simulink model "sistemaUno"  (R2013b)
settings: Solver=ode45  StartTime=0.0  StopTime=100  RelTol=1e-5
settings Model: Creator=juan_  LastModifiedBy=juan_

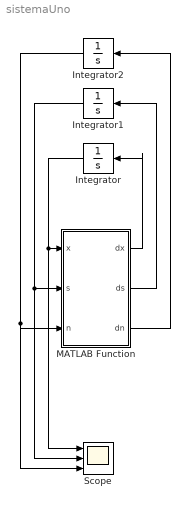
== system sistemaUno ==
  Integrator : Integrator  InitialCondition=1
  Integrator1 : Integrator  InitialCondition=50
  Integrator2 : Integrator  InitialCondition=10
  MATLAB Function : MATLAB Function  TreatAsAtomicUnit=on
  Scope : Scope  NumInputPorts=3
      settings: TimeRange=50  YMin=-5~-5~-5  YMax=5~5~5  SampleInput=on
  wires:
  MATLAB Function/1(dx) -> Integrator/1
  Integrator/1 -> Scope/1, MATLAB Function/1(x)
  MATLAB Function/2(ds) -> Integrator1/1
  MATLAB Function/3(dn) -> Integrator2/1
  Integrator1/1 -> Scope/2, MATLAB Function/2(s)
  Integrator2/1 -> Scope/3, MATLAB Function/3(n)

== matlab function sistemaUno/MATLAB Function ==
  data: x input; dx output; s input; n input; ds output; dn output
function [dx,ds,dn] = fcn(x,s,n)

k1=1/0.45;
k2=0.108;
s_in=50;
n_in=5;
D=0;

x0=1;
s0=50;
n0=10;

mu_max=0.5;
Ks=0.5;
rx=x*mu_max*s/(Ks+s);
rs=-k1*rx;
rn=-k2*rx;

dx= rx+D*(-x);
ds= rs+D*(s_in-s);
dn= rn+D*(n_in-n);
